simulink model "DC"  (R2019a)
settings: Solver=FixedStepAuto  StartTime=0.0  StopTime=300  FixedStep=0.01  RelTol=1e-3
libraries: fuzblock x4
settings Model: Creator=ASUS  LastModifiedBy=ASUS

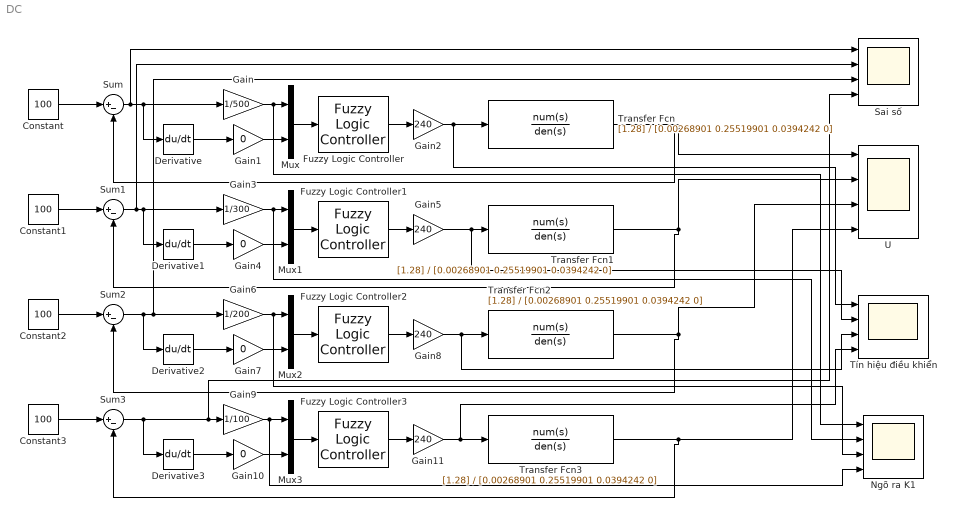
== system DC ==
  Constant{,1..3} (4 alike) : Constant  Value=100
  Derivative{,1..3} (4 alike) : Derivative
  Fuzzy Logic Controller{,1..3} (4 alike) : fuzblock/Fuzzy Logic  Controller  FIS='dongco.fis'  OutputSampleNumber=101  DataType=double  FuzzifiedInputs=off  RuleFiringStrengths=off  RuleOutputs=off  AggregatedOutputs=off  SimulateUsing=Interpreted execution  OutOfRangeInputValueMessage=warning  NoRuleFiredMessage=warning  EmptyOutputFuzzySetMessage=warning
  Gain : Gain  Gain=1/500
  Gain{1,4,7,10} (4 alike) : Gain  Gain=0
  Gain{2,5,8,11} (4 alike) : Gain  Gain=240
  Gain3 : Gain  Gain=1/300
  Gain6 : Gain  Gain=1/200
  Gain9 : Gain  Gain=1/100
  Mux{,1..3} (4 alike) : Mux  Inputs=2
  Ngõ ra K1 : Scope  NumInputPorts=4
  Sai số : Scope  NumInputPorts=4
  Sum{,1..3} (4 alike) : Sum  Inputs=|+-
  Transfer Fcn{,1..3} (4 alike) : TransferFcn  Numerator=[1.28]  Denominator=[0.00268901 0.25519901 0.0394242 0]
  "Tín hiệu điều khiển " : Scope  NumInputPorts=4
  U : Scope  NumInputPorts=4
  wires:
  Derivative/1 -> Gain1/1
  Gain1/1 -> Mux/2
  Gain/1 -> Ngõ ra K1/1, Mux/1
  Mux/1 -> Fuzzy Logic Controller/1
  Fuzzy Logic Controller/1 -> Gain2/1
  Gain2/1 -> "Tín hiệu điều khiển "/1, Transfer Fcn/1
  Transfer Fcn/1 -> Sum/2, U/1
  Sum/1 -> Sai số/1, Derivative/1, Gain/1
  Constant/1 -> Sum/1
  Transfer Fcn1/1 -> Sum1/2, U/2
  Gain4/1 -> Mux1/2
  Derivative1/1 -> Gain4/1
  Gain3/1 -> Ngõ ra K1/2, Mux1/1
  Constant1/1 -> Sum1/1
  Gain5/1 -> "Tín hiệu điều khiển "/2, Transfer Fcn1/1
  Fuzzy Logic Controller1/1 -> Gain5/1
  Mux1/1 -> Fuzzy Logic Controller1/1
  Sum1/1 -> Sai số/2, Derivative1/1, Gain3/1
  Transfer Fcn2/1 -> Sum2/2, U/3
  Gain7/1 -> Mux2/2
  Derivative2/1 -> Gain7/1
  Gain6/1 -> Ngõ ra K1/3, Mux2/1
  Constant2/1 -> Sum2/1
  Gain8/1 -> "Tín hiệu điều khiển "/3, Transfer Fcn2/1
  Fuzzy Logic Controller2/1 -> Gain8/1
  Mux2/1 -> Fuzzy Logic Controller2/1
  Sum2/1 -> Sai số/3, Gain6/1, Derivative2/1
  Transfer Fcn3/1 -> Sum3/2, U/4
  Gain10/1 -> Mux3/2
  Derivative3/1 -> Gain10/1
  Gain9/1 -> Ngõ ra K1/4, Mux3/1
  Constant3/1 -> Sum3/1
  Gain11/1 -> "Tín hiệu điều khiển "/4, Transfer Fcn3/1
  Fuzzy Logic Controller3/1 -> Gain11/1
  Mux3/1 -> Fuzzy Logic Controller3/1
  Sum3/1 -> Sai số/4, Gain9/1, Derivative3/1
